simulink model "EMC_no_hand"  (R2015a)
settings: Solver=ode4  SolverMode=MultiTasking  StartTime=0.0  StopTime=inf  FixedStep=BKIN_STEP_TIME  RelTol=1e-3
StartFcn:
  |  warndlg('Dexterit-E models cannot run under simulation. Please compile your model and run it from within Dexterit-E.');set_param(bdroot,'SimulationCommand','stop')
model workspace (MAT data in the model file):
  BKIN_KINEMATIC_FRAME_SIZE = 400
  BKIN_STEP_TIME = 0.00025
  COLOR = 4
  COL_X = 1
  COL_Y = 2
  E_NO_EVENT = 0
  LOAD_X = 1
  LOAD_Y = 2
  MOVEMENT_DELAY = 3
  PATH_LENGTH = 1
  PATH_PERIOD = 2
  POST_TRIAL_DELAY = 4
  RADIUS = 3
  TRAJECTORY = 1
  TRAJECTORY_TYPE = 2
  TRIAL_END = 3
  TRIAL_MOVEMENT = 2
  TRIAL_RESET = 4
  TRIAL_START = 1
  X_POSITION = 1
  Y_POSITION = 2
  col_x = 1
  col_y = 2
  ANGULAR_THRESHOLD = 5
  GAZE_EXIT = 6
  START_REACHED = 7
  FIXATION_DURATION = 6
  TRACKING_TARGET_ROW = 7
  FEEDBACK_COLOR = 5
  CROSS_LOGICAL_RADIUS = 8
  DETECT_FIXATION = 8
  GAZE_IN_TARGET = 5
  START_STABILIZATION = 9
  HAND_IN_TARGET = 9
  BACKGROUND_LOAD = 10
  DIST_BETWEEN_TRAJ = 11
  STRAIGHT_PAUSE_TIME = 12
libraries: simulink x14, xpcrtudplib x12, xpcutilitieslib x10, xpcobsoletelib x8, slrtlib x2, ethercat x2, General x2, Video x2
(part 4 of 6)

== matlab function EMC_no_hand/DataLogging/Create KINARM Data Subsystem/bitfield ==
  data: motorStatus input; bitfield output
function bitfield = buildBitField(motorStatus)

%the bits are 0=motor enabled, 1=disabled. This logic is 
%attempting to reverse that. 
lowbits = bitand(bitxor(motorStatus(1), 3), 3);
highbits = bitand(bitxor(motorStatus(2), 3), 3);

currentLimitBits = bitand(motorStatus(3), 1) + bitshift(bitand(motorStatus(4), 1), 1) + ...
     bitshift(bitand(motorStatus(5), 1), 2) +  bitshift(bitand(motorStatus(6), 1), 3);

gripBits = bitand(motorStatus(7) ,1) + bitshift(bitand(motorStatus(8), 1), 1);

bitfield = lowbits + bitshift(highbits, 2) + bitshift(currentLimitBits, 4) + bitshift(gripBits, 8);

== matlab function EMC_no_hand/Position function/Main//Start target VCODE2 ==
  data: trialInProgress input; pseudorandom_table input; diagonal_table input; sinusoidal_table input; pathLength input; pathPeriod input; straightPauseTime input; distanceBetweenTrajectories input; trialStartTrigger input; outTargetVCode output size=[1,70]; inTargetVCode input; inTrajectory input; inTrajectoryType input
function outTargetVCode = generateVCode(trialInProgress, pseudorandom_table, diagonal_table, sinusoidal_table, pathLength, pathPeriod, straightPauseTime, distanceBetweenTrajectories, trialStartTrigger, inTargetVCode, inTrajectory, inTrajectoryType)
%#codegen

    %VCode position values (indices (3) and (4)) are in m, whereas all gain
    %values (e.g. A1x) are in cm and position calculations are completed in
    %cm.
    
    %Trajectory Parameter Table Key:
    %Row 1: A1x
    %Row 2: A2x
    %Row 3: Harmonic x
    %Row 4: Phase x (degrees)
    %Row 5: A1y
    %Row 6: A2y
    %Row 7: Harmonic y
    %Row 8: Phase y (degrees)
    
    %Declare and initialize the variable representing the updated VCode
    newTargetVCode = inTargetVCode;
    
    %Amplitude of sine waves: TODO test values
    a = 5;%centimeters
    
    %Declare and initialize persistent variables; which define target
    %position, time clock, and trajectory parameters
    persistent x_offset y_offset targetX targetY targetStartX targetStartY trajectory trajectoryType timeClock parameterTable A1x A2x hx px A1y A2y hy py w numWaves theta rightDirection upDirection pathXLength;
    if isempty(targetX) || isempty(x_offset) || isempty(y_offset) || isempty(targetY) || isempty(trajectory) || isempty(trajectoryType) || isempty(timeClock) || isempty(A1x) || isempty(A2x) || isempty(hx) || isempty(px) || isempty(A1y) || isempty(A2y) || isempty(hy) || isempty(py) || isempty(w) || isempty(numWaves)  || isempty(pathXLength) || isempty(theta) || isempty(rightDirection) || isempty(upDirection)
        targetX = -1;
        targetY = -1;
        x_offset = -1;
        y_offset = -1;
        pathXLength = -1;
        targetStartX = -1;
        targetStartY = -1;
        timeClock = -1;
        parameterTable = -1;
        A1x = -1;
        A2x = -1;
        hx = -1;
        px = -1;
        A1y = -1;
        A2y = -1;
        hy = -1;
        py = -1;
        w = -1;
        numWaves = -1;
        theta = -1;
        rightDirection = -1;
        upDirection = -1;
        trajectoryType = -1;
        trajectory = -1;
    end
    
    %If the trial start trigger is being fired, generate new velocity & starting target positions for the upcoming trial
    if trialStartTrigger == 1
        trajectory = inTrajectory;%Gives the trajectory number within the trajectory type
        trajectoryType = inTrajectoryType;%Pseudorandom, sinusoidal, diagonal, vertical, or horizontal
        timeClock = 0;
        
        %Set trajectory parameter values for pseudorandom trajectories
        if trajectoryType == 1
            targetStartX = inTargetVCode(3) * 100;%convert to cm
            targetStartY = inTargetVCode(4) * 100;%convert to cm
            parameterTable = pseudorandom_table;
            traj_type = ceil(trajectory / 4);
            A1x = parameterTable(1,traj_type);
            A2x = parameterTable(2,traj_type);
            hx = parameterTable(3,traj_type);
            px = parameterTable(4,traj_type);
            A1y = parameterTable(5,traj_type);
            A2y = parameterTable(6,traj_type);
            hy = parameterTable(7,traj_type);
            py = parameterTable(8,traj_type);
            
            %Up/Right direction
            if traj_type < 4
            	upDirection = -1;
            else
                upDirection = 1;
            end
            rightDirection = -1;
            
            %Calculate frequency
            w = 1 / pathPeriod;
            
            x_offset = rightDirection * (A1x + A2x * cosd(-px));
            y_offset = upDirection * (A2y * sind(-py));
            
        %Set trajectory parameter values for sinusoidal trajectories
        elseif trajectoryType == 4
            parameterTable = sinusoidal_table;
            w = parameterTable(1,trajectory) * 0.01;%Frequency: # Full oscillations (waves) per centimeter
            
            %Calculate x distance needed for desired arc length
            x = linspace(0,(1 / w),1000);%TODO is 100 good enough? Probably
            y = a * sin(2*pi*w * x);
            clf = hypot(diff(x),diff(y));
            unit_arclen = sum(clf);
            num_arcs = pathLength / unit_arclen;%pathLength is in cm
            pathXLength = num_arcs / w;%in cm
            rightDirection = parameterTable(2,trajectory);
            upDirection = parameterTable(3,trajectory);
            targetStartX = inTargetVCode(3) * 100;%convert to cm
            targetStartY = inTargetVCode(4) * 100;%convert to cm
            
        %Set trajectory parameter values for straight-line trajectories
        else
            parameterTable = diagonal_table;
            theta = parameterTable(1,trajectory);%angle of diagonal line, ignored in horizontal/vertical
            rightDirection = parameterTable(2,trajectory);
            %upDirection = parameterTable(3,trajectory);
            upDirection = 1;%NOTE: This is a modification for the out-and-back version of the task.
                            %If we revert, uncomment the original
                            %assignment instead.
            offsetNumber = ceil(trajectory / 4) - 3;%returns -2, -1, 0, 1, or 2
            if trajectoryType == 2%diagonal
                if upDirection == 1
                    targetStartX = inTargetVCode(3) * 100;%convert to cm
                    targetStartY = inTargetVCode(4) * 100;%convert to cm
                else
                    targetStartX = inTargetVCode(3) * 100 - rightDirection * 0.5 * pathLength * cosd(theta);%convert to cm
                    targetStartY = inTargetVCode(4) * 100 + 0.5 * pathLength * sind(theta);%convert to cm
                end
            elseif trajectoryType == 3%vertical
                targetStartX = inTargetVCode(3) * 100 + offsetNumber * distanceBetweenTrajectories;%convert to cm
                if upDirection == 1
                    targetStartY = inTargetVCode(4) * 100;%convert to cm
                else
                    targetStartY = inTargetVCode(4) * 100 + (pathLength / 2);%convert to cm
                end
            else%horizontal
                targetStartX = inTargetVCode(3) * 100;%convert to cm
                targetStartY = inTargetVCode(4) * 100 + offsetNumber * distanceBetweenTrajectories;%convert to cm
            end
            
            %Initialize target position coordinates
            targetX = targetStartX;%convert to cm
            targetY = targetStartY;%convert to cm
        end
    end
            
    %If the trial is in progress, update the target position
    if trialInProgress == 1 % The target is displayed
        
        %Set the time value in seconds
        t = timeClock / 4000;%simulation runs at 4 kHz
        
        %Update the position of the target for pseudorandom trajectories
        if trajectoryType == 1
            adjusted_t = t * (1800/pathPeriod);
            targetX = targetStartX - x_offset + rightDirection * (A1x * cosd(w * adjusted_t) + A2x * cosd(hx * w * adjusted_t - px));%Note:
            targetY = targetStartY - y_offset + upDirection * (A1y * sind(w * adjusted_t) + A2y * sind(hy * w * adjusted_t - py));%These calculations are done in degrees.
        elseif trajectoryType == 4 %Update the position of the target for sinusoidal trajectories
            targetX = targetStartX + rightDirection * (t * pathXLength / pathPeriod);%TODO change, assumes path length is the horizontal distance (maybe ok? probably not.)
            targetY = targetStartY + upDirection * (a * sin(2*pi*w * (targetX - targetStartX)));
        elseif trajectoryType == 2 %Update the position of the target for diagonal trajectories
            if (t > ((pathPeriod / 2) - (straightPauseTime / 2))) & (t < ((pathPeriod / 2) + (straightPauseTime / 2))) %pause target
                targetX = targetStartX + rightDirection * (((pathPeriod / 2)-(straightPauseTime/2)) * pathLength * cosd(theta) / pathPeriod);
                targetY = targetStartY + upDirection * (((pathPeriod / 2)-(straightPauseTime/2)) * pathLength * sind(theta) / pathPeriod);
            elseif t < pathPeriod /2
                targetX = targetStartX + rightDirection * (t * pathLength * cosd(theta) / pathPeriod);
                targetY = targetStartY + upDirection * (t * pathLength * sind(theta) / pathPeriod);
            else%"out and back"
                targetX = targetStartX + rightDirection * 0.5 * pathLength * cosd(theta) - rightDirection * ((t-(pathPeriod / 2)) * pathLength * cosd(theta) / pathPeriod);
                targetY = targetStartY + upDirection * 0.5 * pathLength * sind(theta) - upDirection * ((t-(pathPeriod / 2)) * pathLength * sind(theta) / pathPeriod);
            end
        elseif trajectoryType == 3 %Update the position of the target for vertical trajectories
            targetX = targetStartX;
            if (t > ((pathPeriod / 2) - (straightPauseTime / 2))) & (t < ((pathPeriod / 2) + (straightPauseTime / 2))) %pause target
                targetY = targetStartY + upDirection * (((pathPeriod / 2)-(straightPauseTime/2)) * pathLength/ pathPeriod);
            elseif t < pathPeriod /2
                targetY = targetStartY + upDirection * (t * pathLength/ pathPeriod);
            else
                targetY = targetStartY + upDirection * 0.5 * pathLength - upDirection * ((t-(pathPeriod/2)) * pathLength/ pathPeriod);
            end
        elseif trajectoryType == 5 %Update the position of the target for horizontal trajectories
            if (t > ((pathPeriod / 2) - (straightPauseTime / 2))) & (t < ((pathPeriod / 2) + (straightPauseTime / 2))) %pause target
                targetX = targetStartX + rightDirection * (((pathPeriod / 2)-(straightPauseTime/2)) * pathLength/ pathPeriod);
            elseif t < pathPeriod /2
                targetX = targetStartX + rightDirection * (t * pathLength/ pathPeriod);
            else
                targetX = targetStartX + rightDirection * 0.5 * pathLength - rightDirection * ((t-(pathPeriod/2)) * pathLength/ pathPeriod);
            end
            targetY = targetStartY;
        end
        
        %Update the VCODES to reflect the current x and y positions of the target
        newTargetVCode(3) = targetX * 0.01;%convert to meters
        newTargetVCode(4) = targetY * 0.01;%convert to meters
        
        %Update the clock
        timeClock = timeClock + 1;
    end
    outTime = timeClock;
    outTargetVCode = newTargetVCode;
end

== stateflow chart EMC_no_hand/DataLogging/Poll KINARM/createKINData/Calibration_check ==
  state Monitor/
    entry: trigger_calibration = [0, 0];
    state Robot1 [parallel]
      settings: executionOrder=1
      state Init/
      state Calibrated/
      state WaitForOp/
      state Short_wait/
      state Done/
        entry: trigger_calibration(1) = 1;
      (default) -> Monitor.Robot1.Init
      Monitor.Robot1.Init -> Monitor.Robot1.Calibrated : [is_calibrated(1) == 1]
      Monitor.Robot1.Calibrated -> Monitor.Robot1.WaitForOp [order 1] : [system_type == ECAT]
      Monitor.Robot1.Calibrated -> Monitor.Robot1.Done [order 2]
      Monitor.Robot1.WaitForOp -> Monitor.Robot1.Short_wait : [ecat_state == SAFE_OP]
      Monitor.Robot1.Short_wait -> Monitor.Robot1.Done : after(0.001, sec)
    state Robot2 [parallel]
      settings: executionOrder=2
      state Init/
      state Calibrated/
      state WaitForOp/
      state Short_wait/
      state Done/
        entry: trigger_calibration(2) = 1;
      (default) -> Monitor.Robot2.Init
      Monitor.Robot2.Init -> Monitor.Robot2.Calibrated : [is_calibrated(2) == 1]
      Monitor.Robot2.Calibrated -> Monitor.Robot2.WaitForOp [order 1] : [system_type == ECAT]
      Monitor.Robot2.Calibrated -> Monitor.Robot2.Done [order 2]
      Monitor.Robot2.WaitForOp -> Monitor.Robot2.Short_wait : [ecat_state == SAFE_OP]
      Monitor.Robot2.Short_wait -> Monitor.Robot2.Done : after(0.001, sec)
  (default) -> Monitor
  data: is_calibrated input; system_type input; ECAT constant double =2; ecat_state input; SAFE_OP constant double =4; trigger_calibration output

== matlab function EMC_no_hand/DataLogging/monitor torques/current_limits ==
  data: motor_current_limits input; robot_limits output
function robot_limits  = current_limits(motor_current_limits)

robot_limits = [sum(motor_current_limits(1:2)), sum(motor_current_limits(3:4)), sum(motor_current_limits)];

end

== matlab function EMC_no_hand/DataLogging/monitor torques/delay/filter ==
  data: data input; filteredVals output; filterConsts input
function filteredVals  = filter(data, filterConsts)
    %given any number of input values this will filter those values based
    %on a 2nd order Butterworth filter. You will need to get the constants
    %from http://www-users.cs.york.ac.uk/~fisher/mkfilter/trad.html

    persistent rawVelocities filtVelocities
    valueCount = length(data);
    
    if isempty(rawVelocities)
        rawVelocities = zeros(valueCount, 3);
        filtVelocities = zeros(valueCount, 3);
    end    
    
    filteredVals = zeros(1, valueCount);  
    
    %this code is roughly derrived from the example code given when you
    %generate filter constants at: http://www-users.cs.york.ac.uk/~fisher/mkfilter/trad.html
    for n=1:valueCount        
        GAIN = filterConsts(1);
        rawVelocities(n,:) = insertVal(rawVelocities(n,:),  data(n) / GAIN); 
        filtVelocities(n,:) = insertVal(filtVelocities(n,:), 0);        
        filtVelocities(n,3) = filterValue(rawVelocities(n,:), filtVelocities(n,:), filterConsts);        
        filteredVals(n) = filtVelocities(n,3); 
    end
end

function filtVel = filterValue(velocities, filtVelocities, filterConsts)
    %all filter constants from http://www-users.cs.york.ac.uk/~fisher/mkfilter/trad.html
   filtVel = velocities(1) + ...
         velocities(2) * 2.0 + ...
         velocities(3) + ...
         filtVelocities(1) * filterConsts(2) + ...
         filtVelocities(2) * filterConsts(3);
     
    if isnan(filtVel) || isinf(filtVel)
         filtVel = 0;
    end
end

function arr=insertVal(arr, v)
    arr(1) = arr(2);
    arr(2) = arr(3);
    arr(3) = v;
end

== matlab function EMC_no_hand/DataLogging/Create KINARM Data Subsystem/select KINData/MATLAB Function ==
  data: uu input; dd_out output
function dd_out = fcn(uu)
%#codegen

%when you have an int32 or uint32 and you need to send it to Dex this is
%the right way to do it. 

ss = typecast(uu, 'single');
dd_out = double(ss);

== stateflow chart EMC_no_hand/DataLogging/Network Transfer Subsystem/Send Control Machine ==
  state UpdatePacketQueue [parallel]
    settings: executionOrder=1
    state AddPacketToQueue/
    AddPacketToQueue -> (junction 178)
    (junction 178) -> (junction 49) [order 1] : e_data_ready_strobe
        | {
        | // Prepend the data of the new packet in the queue with the packet's index,
        | // a.k.a. "tracking number".
        | packet_index++;
        | packet_queue[2][queue_head] = single(packet_index);
        | //identify the packet version
        | packet_queue[1][queue_head] = -12;
        |
        | // Copy the new packet into the packet_queue. //CopyInput();
        | recordPacket(&packet_queue[j][queue_head], FULL_PACKET_SIZE, ...
        | 	data_in, KINEMATIC_LEN);
        | // Increment the head pointer of the packet_queue for the next packet.
        | queue_head = fmod(queue_head + 1, packet_queue_sz);
        | }
    (junction 178) -> AddPacketToQueue [order 2]
    (default) -> AddPacketToQueue
    (junction 47) -> AddPacketToQueue : {TrackQueueSize();}
    (junction 49) -> (junction 46) [order 2]
    (junction 49) -> (junction 46) [order 1] : [packet_index == max_packet_id]
        | {packet_index = 0;}
    (junction 46) -> (junction 47) [order 2]
    (junction 46) -> (junction 47) [order 1] : [ queue_head == queue_tail]
        | {queue_tail = fmod(queue_tail + 1, packet_queue_sz);}
  note: Packet Queue Versions:
      |
      | -10 - Originals
      | -11 - Added "runID" at [4]
      | -12 - Added CRC
  note: BE-AWARE - packet_queue's definition looks very strange,
      | this is on purpose.
      | Packet_queue is packet_size x 50k. This looks a bit odd and
      | would be wrong in C. However, the way MATLAB generates
      | the C code is to flip the 2 axis to 50k x packet_size. When
      | we used to define the queue as 50K x packet_size, in order
      | to copy a packet would require jumps of 50k for each value
      | read - HIGHLY innefficient. By inverting the axis in the model
      | explorer we save ~30 microseconds per send.
  note: The packed KINEMATIC data is 400 singles long.
      | There is a header of 10 singles at the beginning.
      | Right now we only use 0-5. The remaining singles
      | are "reserved" for future use. Mainly they are in
      | place in case we have more trouble with DEX-3274
      | in the future.
  state SendControlMachine [parallel]
    settings: executionOrder=2
    state Fixed/
      resetUDP = 0;
      state Idle
        // Wait to acquire a new packet to send.
      state SendPacket/
        buildOutputPacket(data_out, &packet_queue[0][queue_tail], FULL_PACKET_SIZE, ...
        queue_size,total_timeouts, runID);
        outstanding_packet_index = data_out[2];
        e_send;
      note: DEX-3274: The send control system here has been
          | updated extensively to account for UDP stack corruption issues.
          | The main areas here that are critical are:
          | 1. e_fast_clk on each transition. This is required in order to ensure that
          | we do not try to send more than one packet in a single time step
          | 2. The UDP reset system. The UDP reset system sees when the
          | queue has grown too large and then forces the UDP port to be reset
          | to clear what is likely corrupt data in the system.
      (default) -> Idle
      (junction 376) -> Idle [order 1] : [queue_head == queue_tail]
      (junction 377) -> (junction 376)
      (junction 376) -> SendPacket [order 2] : [queue_head != queue_tail]
      (junction 378) -> (junction 377) : e_fast_clk[ack_packet_index == outstanding_packet_index]
          | { queue_tail = fmod(queue_tail + 1, packet_queue_sz); }
      Idle -> SendPacket : e_fast_clk[queue_head != queue_tail]
      SendPacket -> (junction 378) [order 2]
      SendPacket -> (junction 379) [order 1] : e_fast_clk[after(10, e_clk)]
      (junction 405) -> SendPacket [order 1] : [is_exam_running == 0]
          | {total_timeouts++;}
      (junction 380) -> SendPacket : {total_timeouts++;}
      (junction 379) -> (junction 405)
      (junction 405) -> (junction 380) [order 2]
    state ResetUDPPort/
      resetUDP = 1;
    (default) -> Fixed
    Fixed -> ResetUDPPort : e_reset_UDP
    ResetUDPPort -> Fixed : after(2, e_fast_clk)
  state TrackQueueSize [function]
    (default) -> (junction 40)
    (junction 40) -> (junction 41) [order 1] : [queue_head < queue_tail]
        | { queue_size = queue_head + packet_queue_sz - queue_tail; }
    (junction 40) -> (junction 41) [order 2] : [queue_head >= queue_tail]
        | { queue_size = queue_head - queue_tail; }
  state FixMonitor [parallel]
    settings: executionOrder=3
    state Fix/
      send(e_reset_UDP, SendControlMachine);
    state NoFix/
    (default) -> NoFix
    NoFix -> Fix : [queue_size > 2500]
    Fix -> NoFix : e_fast_clk[after(1000, e_clk) ]
  data: resetUDP output double =0; data_out output single size=FULL_PACKET_SIZE; data_in input single size=KINEMATIC_LEN; queue_tail local uint32 =0; queue_size output single =0; total_timeouts output single =0; packet_index local uint32 =0; ack_packet_index input uint32; max_packet_id input uint32; runID input single; packet_queue local single size=[FULL_PACKET_SIZE 50000]; packet_queue_sz local double =50000; j local int32; KINEMATIC_LEN constant int32 =400; FULL_PACKET_SIZE constant int32 =410; outstanding_packet_index local double; queue_head local uint32; is_exam_running input double
  events: e_send output FUNCTION_CALL_EVENT; e_data_ready_strobe input RISING_EDGE_EVENT; e_clk input RISING_EDGE_EVENT; e_fast_clk input EITHER_EDGE_EVENT; e_reset_UDP local FUNCTION_CALL_EVENT

== matlab function EMC_no_hand/DataLogging/Network Transfer Subsystem/force strobe/force strobe ==
  data: strobe input; strobe_out output
function strobe_out = fcn(strobe)
%#codegen
% DEX-3234 - it turns out that if we try to send 1 kinematic packet of data
% per UDP packet then the "strobe" from the packet creating sub-system just
% stays high - i.e. always send data. The trouble is that signal is used by
% the Sending state flow diagram and in order to be used as a proper
% stateflow input event the strobe has to change. This code runs at double
% the speed of the packet creating sub system. That allows us to force the
% strobe to zero on alternate steps so that we can properly signal on a true
% strobe going to 1.
persistent counter

if isempty(counter)
    counter = 0;
end

counter = counter + 1;

if mod(counter, 2) == 0
    strobe_out = 0;
    counter = 0;
else
    strobe_out = double(strobe);
end

== matlab function EMC_no_hand/DataLogging/monitor torques/filter ==
  data: data input; filteredVals output; filterConsts input
function filteredVals  = filter(data, filterConsts)
    %given any number of input values this will filter those values based
    %on a 2nd order Butterworth filter. You will need to get the constants
    %from http://www-users.cs.york.ac.uk/~fisher/mkfilter/trad.html

    persistent rawVelocities filtVelocities
    valueCount = length(data);
    
    if isempty(rawVelocities)
        rawVelocities = zeros(valueCount, 3);
        filtVelocities = zeros(valueCount, 3);
    end    
    
    filteredVals = zeros(1, valueCount);  
    
    %this code is roughly derrived from the example code given when you
    %generate filter constants at: http://www-users.cs.york.ac.uk/~fisher/mkfilter/trad.html
    for n=1:valueCount        
        GAIN = filterConsts(1);
        rawVelocities(n,:) = insertVal(rawVelocities(n,:),  data(n) / GAIN); 
        filtVelocities(n,:) = insertVal(filtVelocities(n,:), 0);        
        filtVelocities(n,3) = filterValue(rawVelocities(n,:), filtVelocities(n,:), filterConsts);        
        filteredVals(n) = filtVelocities(n,3); 
    end
end

function filtVel = filterValue(velocities, filtVelocities, filterConsts)
    %all filter constants from http://www-users.cs.york.ac.uk/~fisher/mkfilter/trad.html
   filtVel = velocities(1) + ...
         velocities(2) * 2.0 + ...
         velocities(3) + ...
         filtVelocities(1) * filterConsts(2) + ...
         filtVelocities(2) * filterConsts(3);
     
    if isnan(filtVel) || isinf(filtVel)
         filtVel = 0;
    end
end

function arr=insertVal(arr, v)
    arr(1) = arr(2);
    arr(2) = arr(3);
    arr(3) = v;
end

== matlab function EMC_no_hand/DataLogging/Receive_Gaze/Create timestamp ==
  data: time_in input; timestamp_out output; start_time_out output
function [timestamp_out, start_time_out] = fcn(time_in)

persistent start_time
persistent last_time

if isempty(start_time)
   start_time = -1;
end

if isempty(last_time)
    last_time = -1;
end

if start_time == -1 && time_in ~= 0
    start_time = time_in;
end

%if the clock has flipped over then in order to get the time
%right this will add the time before the flip to the current time.
if time_in < start_time
    start_time = -(last_time - start_time);
end

timestamp_out = (time_in - start_time) / 1000.0;
last_time = time_in;
start_time_out = start_time;

== matlab function EMC_no_hand/DataLogging/Receive_Gaze/Embedded MATLAB Function1 ==
  data: input input; pupil_area_PIXELS input; tracking_status input; tracking_available input; camtheta input; camera_GLOBAL input; focal_length input; gazeXYCalculated output; head_data input; pupil_area_GLOBAL output; gaze_unit_vector_GLOBAL output; pupil_GLOBAL output; target_GLOBAL output
function [gazeXYCalculated, pupil_area_GLOBAL, gaze_unit_vector_GLOBAL, pupil_GLOBAL, target_GLOBAL] = fcn(input, pupil_area_PIXELS, tracking_status, tracking_available, camtheta,camera_GLOBAL, focal_length, head_data)

% The following are some details on the Eyelink camera
EL_target_distance_scaling_factor = 10000;					%target distance is reported by Eyelink in 1/10 of mm units
EL_pix_per_mm = 200;										%there are 200 pixels/mm on the Eyelink 1000 camera sensor

raw_pupil = [input(1) input(2)];
href = [input(3); input(4); 0];
target_distance_in = head_data(3);
%%%%%%%%%%%%%%%%%%%%%%%%%%%%%%%%%%
%% Tarkesh
target_position_in = head_data(1:2);
%%%%%%%%%%%%%%%%%%%%%%%%%%%%%%%%%%%%%%
target_distance = target_distance_in / EL_target_distance_scaling_factor;		% distance of the target from the camera (m)

%if there is a blink or other problem then send out errors. C3D file does not like NaN, so we output -100.
if tracking_status == 4 || tracking_available == 0 || (href(1) == 0 && href(2) == 0) || (raw_pupil(1) == -32768 && raw_pupil(2) == -32768)
    gazeXYCalculated = [-100; -100];
	pupil_area_GLOBAL = -100;
    gaze_unit_vector_GLOBAL = [-100; -100; -100];
    pupil_GLOBAL = [-100; -100; -100];
    target_GLOBAL = [-100; -100; -100];
    return
end

[Rx Ry Rz] = calc_R_from_angles(camtheta(1), camtheta(2), 0);
R_CMRA2GLBL = Rx * Ry;
%R_GLBL2CMRA = R_CMRA2GLBL';

%camera_GLOBAL_Trans = camera_GLOBAL';
pupil_XY_Sensor = convertPupilToSensor(raw_pupil(1), raw_pupil(2), EL_pix_per_mm);
[gaze_GLOBAL, pupil_GLOBAL] = calc_GAZE(pupil_XY_Sensor, target_distance, href, focal_length, camera_GLOBAL, R_CMRA2GLBL);
gazeXYCalculated = gaze_GLOBAL(1:2);

%%%%%%%%%%%%%%%%%%%%%%%%%%5
%% Tarkesh
target_XY_Sesor = convertPupilToSensor(target_position_in(1), target_position_in(2), EL_pix_per_mm);
[~, target_GLOBAL] = calc_GAZE(target_XY_Sesor, target_distance, href, focal_length, camera_GLOBAL, R_CMRA2GLBL);
%%%%%%%%%%%%%%%%%%%%%%%%%%

%%convert the pupil area from pixels on the sensor, to m^2, correcting for camera and gaze angle
% pupil area on the camera sensor, in m^2
pupil_area_SENSOR = pupil_area_PIXELS / ( (EL_pix_per_mm * 1000 ) ^ 2);		

% pupil area in the global workspace, projected onto a plane parallel to the camera sensor in m^2
pupil_area_GLOBAL_projection = pupil_area_SENSOR * (target_distance / focal_length) ^ 2; 

% create a unit vector that is normal to the camera sensor, in GLOBAL coordinates
sensor_unit_vector_GLOBAL = R_CMRA2GLBL * [0; 0; 1];

% create a unit vector for the subject's gaze
gaze_vector_GLOBAL = pupil_GLOBAL - gaze_GLOBAL;
gaze_unit_vector_GLOBAL = gaze_vector_GLOBAL / norm(gaze_vector_GLOBAL);

% calculate the cosine of the angle between the unit vectors for gaze and the camera sensor
cos_gaze_camera_angle = dot(sensor_unit_vector_GLOBAL, gaze_unit_vector_GLOBAL); 

% correct the pupil area to account for the angle of the eye relative to the camera sensor plane
% We assume that the pupil is circular. In the plane formed by the two vectors, the distance needs 
% to be scaled by cos(theta). In the perpendicular plane, there is no scaling. Hence we do NOT 
% square the cos(theta) and the area is only corrected for by 1 / cos(theta). 
pupil_area_GLOBAL = pupil_area_GLOBAL_projection / cos_gaze_camera_angle;

% % % % For testing
% % % gaze_camera_angle  = acos(cos_gaze_camera_angle) * 180/pi();
% % % HREF_angle = atan2( norm(href), 15000) * 180 / pi();
% % % testing = [pupil_area_SENSOR*1e6, pupil_area_GLOBAL_projection*1e6, pupil_area_GLOBAL*1e6, gaze_camera_angle, HREF_angle, cos_gaze_camera_angle];
% % % testing2 = [sensor_unit_vector_GLOBAL; gaze_unit_vector_GLOBAL];



%% Functions
function [gaze_est_GLOBAL, pupil_GLOBAL] = calc_GAZE(pupil_SENSOR, target_distance, HREF_HREF, focal_length, camera_GLOBAL, R_CMRA2GLBL)
    % This function estimates GAZE based on data from the Eyelink.  To be used
    % during 'running' of a task. 

    % Convert pupil location from Eyelink sensor frame to camera reference
    % frame with camera at origin and rotated to camera's angle (W-axis along
    % camera's point of view)  
    pupil_CAMERA = [pupil_SENSOR * target_distance / focal_length; target_distance];
    pupil_distance = norm(pupil_CAMERA);

    % Rotation matrix to convert from HREF coordinates to camera coordinates.
    % HREF z-axis is defined as ray from camera to pupil.
    R_HREF2CMRA = calc_R_from_vectors(pupil_CAMERA, [0; 0; 1]);

    % Convert the HREF from HREF coordinates to canera coordinates.  Scale,
    % then rotate. 
    HREF_CAMERA = R_HREF2CMRA * (HREF_HREF * pupil_distance / 15000);

    % Then convert pupil and HREF locations from camera frame to global frame
    % by rotating and then shifting origins. 
    pupil_GLOBAL = R_CMRA2GLBL * pupil_CAMERA + camera_GLOBAL';
    HREF_GLOBAL = R_CMRA2GLBL * HREF_CAMERA + camera_GLOBAL';

    % Find intersection of gaze_ray (from pupil to HREF) with the subject_display plane
    norm_vector = [0; 0; 1];		% In the KINARM VR setup, the Z-axis is defined as normal to the subject display
    point_on_plane = [0; 0; 0];		% In the KINARM VR setup, the origin is defined as on the subject display plane

    % display([pupil_GLOBAL HREF_GLOBAL])
    gaze_est_GLOBAL = plane_line_intersect(norm_vector, point_on_plane, pupil_GLOBAL, HREF_GLOBAL);

function pupil_XY_Sensor = convertPupilToSensor(pupilX, pupilY, pix_per_mm)
%         Returns the projection of the pupil on the camera sensor in meters, based on inputs in some raw unit (not pixels)

    % the following constants are from Jiye, email Nov 7, 2011
    LEFTDROP = 32;				%pixels dropped at left of sensor
    TOPDROP = 48;				%lines dropped at top of sensor
    const_x = 7*176;			%no idea what this is.  Maybe number of pixels???
    const_y = 4*184 + 188;		%no idea what this is.  Maybe number of pixels???

    % from Jiye. Not sure excatly what they are (probably camera center in pixels)
    cam_rot_cx = const_x / 2 + LEFTDROP;			
    cam_rot_cy = const_y / 2 +TOPDROP;

    hor = 30000;
    lor = -30000;
    hr = 0.9;
    lr = 0.1;
    ld = 50;
    hdx = 1200;		%hmmm almost same as const_x, which is 1232
    hdy = 920;		%hmmm almost same as const_y, which is 924

    scx = (hor-lor) / (hdx - ld) / (hr-lr);
    ofx = lor - (ld + (hdx - ld) * lr )* scx;

    scy = (hor-lor) / (hdy - ld) / (hr-lr);
    ofy = lor - (ld + (hdy - ld) * lr )* scy;

    % calculate the pupil in camera sensor coordinates (pixels)
    px = (pupilX - ofx) / scx;
    py = (pupilY - ofy) / scy;

    ppl_mmX = - ( (cam_rot_cx - px) / pix_per_mm );
    ppl_mmY =   ( (cam_rot_cy - py) / pix_per_mm );

    pupil_XY_Sensor = [ppl_mmX / 1000; ppl_mmY / 1000];
    
function [Rx Ry Rz] = calc_R_from_angles(xrot, yrot, zrot)
    % This function creates the three rotation matrices for rotations about the
    % x, y and z axes.  Input rotations are in degrees.

    xrot = xrot/180*pi;		%convert to radians
    yrot = yrot/180*pi;		%convert to radians
    zrot = zrot/180*pi;		%convert to radians
    Rx = [1 0 0; 0 cos(xrot) -sin(xrot); 0 sin(xrot) cos(xrot)]; 
    Ry = [cos(yrot) 0 sin(yrot); 0 1 0; -sin(yrot) 0 cos(yrot)]; 
    Rz = [cos(zrot) -sin(zrot) 0; sin(zrot) cos(zrot) 0 ; 0 0 1]; 

    
function R = calc_R_from_vectors(v1, v2)
    % This function calculates a rotation matrix, given two vectors, such that
    % the rotation matrix will rotate from v1 to v2.

    rot_axis = cross(v2, v1);			%axis that is perpendicular to the two vectors

    % If either of the vectors v1 or v2 is = [0 0 0], or if they are parallel
    % (i.e. norm(rot_axis) == 0), then there is no rotation.  But math errors
    % will occur, so we need to check for these cases.   
    if (norm(v1) == 0) || (norm(v2) == 0)	|| (norm(rot_axis) == 0)
        R = eye(3);																%identity matrix results in no rotation
    else
        rot_angle = asin( norm(rot_axis) / norm(v1) / norm(v2) );				%angle of rotation about rot_axis
        n = rot_axis / norm(rot_axis);											%normalize to get a unit vector for the rotation
        n_cross_product_matrix = [ 0 -n(3) n(2); n(3) 0 -n(1); -n(2) n(1) 0];	%def'n of cross product matrix
        cosA = cos(rot_angle);
        sinA = sin(rot_angle);
        R = eye(3) * cosA + sinA * n_cross_product_matrix + (1 - cosA) * (n * n');
    % 	display(rot_angle);
    end


function I = plane_line_intersect(n,V0,P0,P1)
    %plane_line_intersect computes the intersection of a plane and a segment(or
    %a straight line)
    % Inputs: 
    %       n: normal vector of the Plane 
    %       V0: any point that belongs to the Plane 
    %       P0: end point 1 of the segment P0P1
    %       P1:  end point 2 of the segment P0P1
    %
    %Outputs:
    %      I    is the point of interection 
    %     Check is (DELETED AND NOT USED HERE) an indicator:
    %      0 => disjoint (no intersection)
    %      1 => the plane intersects P0P1 in the unique point I
    %      2 => the segment lies in the plane
    %      3=>the intersection lies outside the segment P0P1
    %
    % Example:
    % Determine the intersection of following the plane x+y+z+3=0 with the segment P0P1:
    % The plane is represented by the normal vector n=[1 1 1]
    % and an arbitrary point that lies on the plane, ex: V0=[1 1 -5]
    % The segment is represented by the following two points
    % P0=[-5 1 -1]
    %P1=[1 2 3]   
    % [I,check]=plane_line_intersect([1 1 1],[1 1 -5],[-5 1 -1],[1 2 3]);

    %This function is written by :
    %                             Nassim Khaled
    %                             Wayne State University
    %                             Research Assistant and Phd candidate
    %If you have any comments or face any problems, please feel free to leave
    %your comments and i will try to reply to you as fast as possible.

    I=[0; 0; 0];
    u = P1-P0;
    w = P0 - V0;
    D = dot(n,u);
    N = -dot(n,w);
    check=0;
    if abs(D) < 10^-7        % The segment is parallel to plane
            if N == 0           % The segment lies in plane
                check=2;
                return
            else
                check=0;       %no intersection
                return
            end
    end

    %compute the intersection parameter
    sI = N / D;
    I = P0+ sI.*u;

== matlab function EMC_no_hand/DataLogging/Receive_Gaze/clean_packet ==
  data: pack_in input; pack_out output; len_out output; len_in input
function [pack_out, len_out] = clean_packet(pack_in, len_in)

%for some reason, during calibration we can get very large packets that 
%blow up the c code for parsing the packets. If we get a large packet
%we can ignore it.

if len_in < 512
    pack_out = pack_in;
    len_out = len_in;
else
    pack_out = zeros(512, 1, 'uint8');
    len_out = int32(0);
end

== matlab function EMC_no_hand/DataLogging/Receive_Gaze/convert to seconds2 ==
  data: event_data input; event_data_out output; start_time input; eyelink_timestamp input
function event_data_out = fcn(event_data, start_time, eyelink_timestamp)

persistent last_timestamp

if isempty(last_timestamp)
	last_timestamp = uint32(0);
end

%DEX-3313 if eyelink has stopped sending us data then we should not flood
%Dex with events.
if last_timestamp == eyelink_timestamp
	event_data_out = [0; 0; 0];
	return
end

last_timestamp = eyelink_timestamp;
event_data_out = event_data;

if event_data(1) ~= 0
    event_data_out(2) = (event_data(2) - start_time) / 1000.0;
    event_data_out(3) = (event_data(3) - start_time) / 1000.0;
end

== matlab function EMC_no_hand/DataLogging/Poll Force Plates/plate1/parse packet 1 ==
  data: packet input; forces output; moments output; timer output; calibration input; gain input; ain_slope input; ain_offset input; orientation input; zero_voltage input
function [forces, moments, timer] = fcn(packet, calibration, gain, ain_slope, ain_offset, orientation, zero_voltage)
    %This pulls voltages and timer infomation from the packet we got back from
    %the lab jack.
    
    voltages = zeros(1, 8);
    timers = zeros(1, 3);
    
    for n = 1:8
        bits = readUShort(packet, 13 + ((n - 1)*2));
        voltages(n) = binaryToCalibratedAnalogVoltage(bits, ain_slope, ain_offset);
    end
    
    for n = 1:3
        timers(n) = readUInt(packet, 53 + ((n - 1)*4));
    end
    
    %convert the time stamp to a time in seconds.
    timer = timers(1) / 750000.0; 
    
    %all voltages are between -2.5 to 2.5, here we are normalizeing what we read to zero.
    voltages = voltages - zero_voltage;
    voltages = voltages(1:8); % only the first 8 channels matter.
    
    %using the calibration matrix we convert the to the forces and moments
    values = calibration * (voltages / gain)';
    forces = values(1:3);
    moments = values(4:6);
    
	%reverse the Z force to get it into global coordinates.
	forces(3) = -forces(3);
	
	%considering the positions of the cables push all measures into global coordinates
    if orientation == 0
        forces(2) = -forces(2);
        moments(2) = -moments(2);
    elseif orientation == 90
        y = forces(2);
        forces(2) = -forces(1);
        forces(1) = -y;

        y = moments(2);
        moments(2) = -moments(1);
        moments(1) = -y;
	elseif orientation == 180
        forces(1) = -forces(1);        
        moments(1) = -moments(1);        
    elseif orientation == 270
        y = forces(2);
        forces(2) = forces(1);
        forces(1) = y;

		y = moments(2);
        moments(2) = moments(1);
        moments(1) = y;
    end
end

function val = readUShort(data, offset)
    p1 = uint32(data(offset));
    p2 = uint32(data(offset + 1));
    val = double(p1 + (p2 * 256));
end

function val = readUInt(data, offset)
    p1 = uint32(data(offset));
    p2 = uint32(data(offset + 1));
    p3 = uint32(data(offset + 2));
    p4 = uint32(data(offset + 3));
    val = double(p1 + (p2 * 256) + (p3 * 2^16) + (p4 * 2^24));
end

function voltage = binaryToCalibratedAnalogVoltage(bits, ain_slope, ain_offset)
    voltage = (bits * ain_slope) + ain_offset;
end

== matlab function EMC_no_hand/DataLogging/Poll Force Plates/plate2/parse packet 1 ==
  data: packet input; forces output; moments output; timer output; calibration input; gain input; ain_slope input; ain_offset input; orientation input; zero_voltage input
function [forces, moments, timer] = fcn(packet, calibration, gain, ain_slope, ain_offset, orientation, zero_voltage)
    %This pulls voltages and timer infomation from the packet we got back from
    %the lab jack.
    
    voltages = zeros(1, 8);
    timers = zeros(1, 3);

    for n = 1:8
        bits = readUShort(packet, 13 + ((n - 1)*2));
        voltages(n) = binaryToCalibratedAnalogVoltage(bits, ain_slope, ain_offset);
    end
    
    for n = 1:3
        timers(n) = readUInt(packet, 53 + ((n - 1)*4));
    end
    
    %convert the time stamp to a time in seconds.
    timer = timers(1) / 750000.0; 
    
    %all voltages are between -2.5 to 2.5, here we are normalizeing what we read to zero.
    voltages = voltages - zero_voltage;
    voltages = voltages(1:8); % only the first 8 channels matter.
    
    %using the calibration matrix we convert the to the forces and moments
    values = calibration * (voltages / gain)';
    forces = values(1:3);
    moments = values(4:6);
    
	%reverse the Z force to get it into global coordinates.
	forces(3) = -forces(3);

	%considering the positions of the cables push all measures into global coordinates
    if orientation == 0
        forces(2) = -forces(2);
        moments(2) = -moments(2);
    elseif orientation == 90
        y = forces(2);
        forces(2) = -forces(1);
        forces(1) = -y;

        y = moments(2);
        moments(2) = -moments(1);
        moments(1) = -y;
	elseif orientation == 180
        forces(1) = -forces(1);        
        moments(1) = -moments(1);        
    elseif orientation == 270
        y = forces(2);
        forces(2) = forces(1);
        forces(1) = y;

		y = moments(2);
        moments(2) = moments(1);
        moments(1) = y;
    end
end

function val = readUShort(data, offset)
    p1 = uint32(data(offset));
    p2 = uint32(data(offset + 1));
    val = double(p1 + (p2 * 256));
end

function val = readUInt(data, offset)
    p1 = uint32(data(offset));
    p2 = uint32(data(offset + 1));
    p3 = uint32(data(offset + 2));
    p4 = uint32(data(offset + 3));
    val = double(p1 + (p2 * 256) + (p3 * 2^16) + (p4 * 2^24));
end

function voltage = binaryToCalibratedAnalogVoltage(bits, ain_slope, ain_offset)
    voltage = (bits * ain_slope) + ain_offset;
end

== matlab function EMC_no_hand/DataLogging/Poll KINARM/Force Sensor Control/Force Sensor 1 Subsystem/Create timestamp ==
  data: times_in input; timestamp_out output
function timestamp_out = fcn(times_in)

persistent start_time
persistent last_time

if isempty(start_time)
   start_time = uint32(0);
end

if isempty(last_time)
    last_time = uint32(0);
end

if start_time == 0 && times_in(2) > 0
    start_time = times_in(2);
end

if times_in(2) < start_time
    start_time = -(last_time - start_time);
end

%F/T sensor clock runs at 7Khz according to the manual,
%using a 32 bit integer for this gives about 7 days before it will roll
%over. This means we need to account for roll overs in order to make
%analysis sane.
timestamp_out = double(times_in(2) - start_time) / 7000.0;
last_time = times_in(2);

== matlab function EMC_no_hand/DataLogging/Poll KINARM/Force Sensor Control/Force Sensor 2 Subsystem/Create timestamp ==
  data: times_in input; timestamp_out output
function timestamp_out = fcn(times_in)

persistent start_time
persistent last_time

if isempty(start_time)
   start_time = uint32(0);
end

if isempty(last_time)
    last_time = uint32(0);
end

if start_time == 0 && times_in(2) > 0
    start_time = times_in(2);
end

if times_in(2) < start_time
    start_time = -(last_time - start_time);
end

%F/T sensor clock runs at 7Khz according to the manual,
%using a 32 bit integer for this gives about 7 days before it will roll
%over. This means we need to account for roll overs in order to make
%analysis sane.
timestamp_out = double(times_in(2) - start_time) / 7000.0;
last_time = times_in(2);

== matlab function EMC_no_hand/DataLogging/Poll KINARM/PMAC Subsystem/read_pmac/DPRAM Access Subsystem/TypeCast ==
  data: u input; y output
function y = fcn(u)

% EML determines output class and size based on first usage
% for some reason the typecast is not setting it correctly, so we 
% explicitly define it first.
y = single(0);

% in order for the typecast to work, both temp and y must be 32 bit
temp = cast(u, 'uint32');
y = typecast(temp, 'single');

== matlab function EMC_no_hand/DataLogging/Poll KINARM/PMAC Subsystem/read_pmac/Monitor_status ==
  data: status_data input; servo_counter input; robotCount input; force_scale output; plcc_version input
function force_scale = monitor_system_status(status_data, servo_counter, robotCount, plcc_version)

persistent no_update_count;
persistent last_servo_counter;

if isempty(no_update_count)
   no_update_count = 0;
end

if isempty(last_servo_counter)
    last_servo_counter = uint32(0);
end

pmac_fault_state = uint32(status_data(2));
plcc_switch = status_data(3);
force_scale = 1;

%plcc versions >1000 are custom
if plcc_version >= 6.0 && plcc_version < 1000
    %if the task is running and the servo amp counter is not
    if plcc_switch == 4.0 && last_servo_counter == servo_counter
        no_update_count = no_update_count + 1;    
        %after 5 cycles with the counter not running we should kill forces.
        if no_update_count >= 5
            force_scale = 0;
        end
    else
        no_update_count = 0;
    end
    last_servo_counter = servo_counter; 
end

%plcc versions >1000 are custom
if plcc_version >= 7.0 && plcc_version < 1000
    %if it is unilateral and the robot state is faulted then kill the forces
    if robotCount == 1 && bitand(pmac_fault_state, 1) == 1
        force_scale = 0;
    %if the system is bilateral and either robot is faulted, kill forces.
    elseif robotCount == 2 && bitand(pmac_fault_state, 3) ~= 0
        force_scale = 0;
    end
end

if plcc_version == 0
    force_scale = 0;
end
